simulink model "DrvStCallerForTest"  (R2018b)
settings: Solver=FixedStepDiscrete  StartTime=0.0  StopTime=10.0  RelTol=1e-3
undefined symbols (not defined in the file): DrvStFtCtrl_Cal, DrvStFtHolderChk_Cal, DrvStFtIsPosChk_Cal, DrvStFtTrgtPosSelc_Cal, DrvStRclCmdSrvCal_Cal
settings Model: Creator=sn2xws  LastModifiedBy=sn2xws
settings DataIOCC: SaveFormat=StructureWithTime
settings OptimizationCC: DefaultParameterBehavior=Inlined  EnhancedBackFolding=on  PassReuseOutputArgsAs=Individual arguments  ZeroExternalMemoryAtStartup=off  ZeroInternalMemoryAtStartup=off  OptimizeBlockOrder=speed  DifferentSizesBufferReuse=on  OptimizationCustomize=off
settings DebuggingCC: ParameterTunabilityLossMsg=error
settings SFSimCC: MATLABDynamicMemAlloc=off
settings RTWCC: SystemTargetFile=autosar.tlc  GenCodeOnly=on  TemplateMakefile=ert_default_tmf  Description=AUTOSAR  GenerateReport=on  IncludeHyperlinkInReport=on  LaunchReport=on  GenerateTraceInfo=on  GenerateTraceReport=on  GenerateTraceReportSl=on  GenerateTraceReportSf=on  GenerateTraceReportEml=on  GenerateCodeMetricsReport=on
settings CodeAppCC: ForceParamTrailComments=on  IgnoreCustomStorageClasses=off  OperatorAnnotations=on  SimulinkDataObjDesc=on  SFDataObjDesc=on  InsertBlockDesc=on
settings STFCustomTargetCC: TargetLangStandard=C99 (ISO)  MultiwordLength=256  ParMdlRefBuildCompliant=on  CompOptLevelCompliant=on  IncludeMdlTerminateFcn=off  CombineOutputUpdateFcns=on  SuppressErrorStatus=on  ERTCustomFileBanners=on  SupportNonFinite=off  SupportComplex=off  SupportContinuousTime=off  SupportNonInlinedSFcns=off  RemoveResetFunc=on  MATLABClassNameForMDSCustomization=Simulink.SoftwareTarget.ERTCustomization  AutosarCompliant=on  UseToolchainInfoCompliant=on  LookupTableObjectStructAxisOrder=2,1,3,4,...  LUTObjectStructOrderEvenSpacing=Size,Table,Breakpoints  SystemTargetFile=autosar.tlc
settings ERTTargetCC: TargetLangStandard=C99 (ISO)  ConcurrentExecutionCompliant=off  IncludeMdlTerminateFcn=off  SuppressErrorStatus=on  SupportNonFinite=off  SupportComplex=off  ModelStepFunctionPrototypeControlCompliant=off  CPPClassGenCompliant=off  AutosarCompliant=on  LookupTableObjectStructAxisOrder=2,1,3,4,...  LUTObjectStructOrderEvenSpacing=Size,Table,Breakpoints  InlinedParameterPlacement=NonHierarchical  ERTCustomFileTemplate=example_file_process.tlc  ERTFilePackagingFormat=Compact

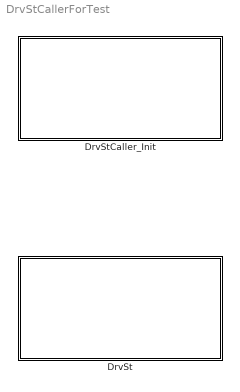
== system DrvStCallerForTest ==
  DrvSt : Subsystem
  DrvStCaller_Init : Subsystem

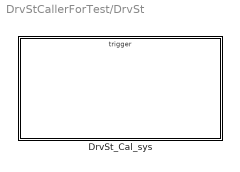
== system DrvStCallerForTest/DrvSt ==
  DrvSt_Cal_sys : Subsystem

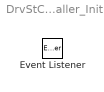
== system DrvStCallerForTest/DrvStCaller_Init ==
  Event Listener : EventListener  EventName=reset

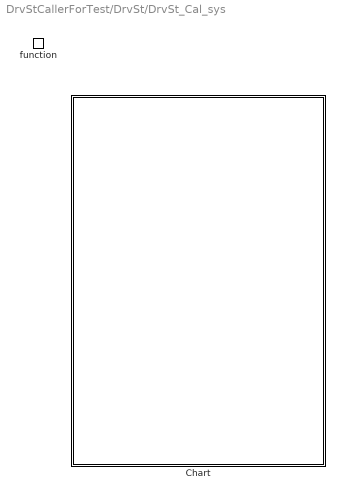
== system DrvStCallerForTest/DrvSt/DrvSt_Cal_sys ==
  function : TriggerPort  TriggerType=function-call  IsSimulinkFunction=on  FunctionName=DrvSt_Cal  VariantControl=(inherit)
  Chart : Stateflow chart  TreatAsAtomicUnit=on

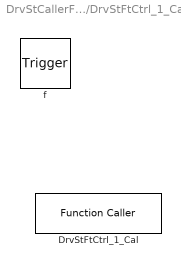
== system DrvStCallerForTest/DrvSt/DrvSt_Cal_sys/Chart/DrvStFtCtrl_1_Cal ==
  f : TriggerPort  TriggerType=function-call  VariantControl=(inherit)
      settings: CopyFcn=Stateflow.SLINSF.SimulinkMan.removeBlockPreDeleteFcn  PreDeleteFcn=Stateflow.SLINSF.SimulinkMan.unsafePredeleteFcn
  DrvStFtCtrl_1_Cal : FunctionCaller  FunctionPrototype=DrvStFtCtrl_Cal()

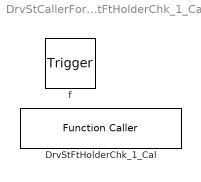
== system DrvStCallerForTest/DrvSt/DrvSt_Cal_sys/Chart/DrvStFtHolderChk_1_Cal ==
  f : TriggerPort  TriggerType=function-call  VariantControl=(inherit)
      settings: CopyFcn=Stateflow.SLINSF.SimulinkMan.removeBlockPreDeleteFcn  PreDeleteFcn=Stateflow.SLINSF.SimulinkMan.unsafePredeleteFcn
  DrvStFtHolderChk_1_Cal : FunctionCaller  FunctionPrototype=DrvStFtHolderChk_Cal()

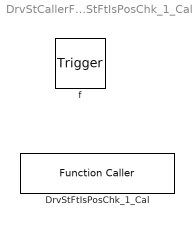
== system DrvStCallerForTest/DrvSt/DrvSt_Cal_sys/Chart/DrvStFtIsPosChk_1_Cal ==
  f : TriggerPort  TriggerType=function-call  VariantControl=(inherit)
      settings: CopyFcn=Stateflow.SLINSF.SimulinkMan.removeBlockPreDeleteFcn  PreDeleteFcn=Stateflow.SLINSF.SimulinkMan.unsafePredeleteFcn
  DrvStFtIsPosChk_1_Cal : FunctionCaller  FunctionPrototype=DrvStFtIsPosChk_Cal()

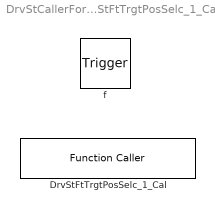
== system DrvStCallerForTest/DrvSt/DrvSt_Cal_sys/Chart/DrvStFtTrgtPosSelc_1_Cal ==
  f : TriggerPort  TriggerType=function-call  VariantControl=(inherit)
      settings: CopyFcn=Stateflow.SLINSF.SimulinkMan.removeBlockPreDeleteFcn  PreDeleteFcn=Stateflow.SLINSF.SimulinkMan.unsafePredeleteFcn
  DrvStFtTrgtPosSelc_1_Cal : FunctionCaller  FunctionPrototype=DrvStFtTrgtPosSelc_Cal()

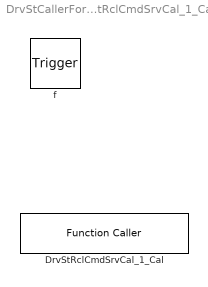
== system DrvStCallerForTest/DrvSt/DrvSt_Cal_sys/Chart/DrvStRclCmdSrvCal_1_Cal ==
  f : TriggerPort  TriggerType=function-call  VariantControl=(inherit)
      settings: CopyFcn=Stateflow.SLINSF.SimulinkMan.removeBlockPreDeleteFcn  PreDeleteFcn=Stateflow.SLINSF.SimulinkMan.unsafePredeleteFcn
  DrvStRclCmdSrvCal_1_Cal : FunctionCaller  FunctionPrototype=DrvStRclCmdSrvCal_Cal()

== stateflow chart DrvStCallerForTest/DrvSt/DrvSt_Cal_sys/Chart ==
  state DrvStFtTrgtPosSelc_1_Cal [function]
  state DrvStFtIsPosChk_1_Cal [function]
  state DrvStFtHolderChk_1_Cal [function]
  state DrvStFtCtrl_1_Cal [function]
  state DrvStRclCmdSrvCal_1_Cal [function]
  (default) -> (junction 1)
  (junction 1) -> (junction 3) : {
      | DrvStFtTrgtPosSelc_1_Cal();
      | DrvStFtIsPosChk_1_Cal();
      | DrvStFtHolderChk_1_Cal();
      | DrvStFtCtrl_1_Cal();
      | DrvStRclCmdSrvCal_1_Cal();
      | }
